simulink model "servolib"  (R2016a)
settings: Solver=VariableStepAuto  StartTime=0.0  StopTime=10.0  MaxStep=.01  RelTol=1e-3
settings Model: SimulationMode=external  Creator=jordan  LastModifiedBy=jordan

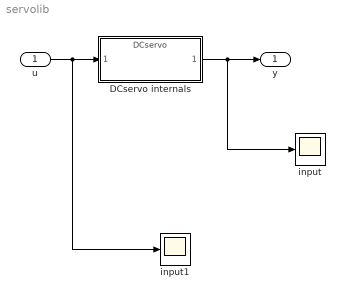
== system servolib ==
  u : Inport
  DCservo internals : ModelReference  ModelNameDialog=DCservo.slxp  ModelReferenceVersion=1.89  CopyOfModelProtected=on
  input : Scope
  input1 : Scope
  y : Outport
  wires:
  DCservo internals/1 -> input/1, y/1
  u/1 -> input1/1, DCservo internals/1
